simulink model "precisionLanding"  (R2021b)
settings: Solver=VariableStepAuto  StartTime=0.0  StopTime=10.0  RelTol=1e-3
values from neighbouring files (symbols this model uses):
  alpha0 = 0.01    [forces_moments.m]    (also in forces_moments_testing.m; omegaController.m; precisionLanding.m)
  D = diag([0 k1*k3 k4/d])    [airspeedController.m]    (also in forces_moments.m; forces_moments_testing.m; precisionLanding.m)
  G = [sin(alpha) 0 -cos(alpha);-cos(alpha)*tan(beta) 1 -sin(alpha)*tan(beta);         cos(alpha)/cos(beta) 0 sin(alpha)/cos(beta)]    [forces_moments.m]    (also in forces_moments_testing.m; precisionLanding.m = [sin(alpha) 0 -cos(alpha);-cos(alpha)*tan(beta) 1 -sin(alpha)
  gama = 1    [airspeedController.m]    (also in forces_moments.m; forces_moments_testing.m; precisionLanding.m)
  k_VI = 0.8    [airspeedController.m]    (also in forces_moments.m; forces_moments_testing.m; main_precision_landing.m; precisionLanding.m)
  k_VP = 0.5    [airspeedController.m]    (also in forces_moments.m; forces_moments_testing.m; main_precision_landing.m; precisionLanding.m)
  Maabb = [P.C_ell_beta 0; 0 P.C_m_alpha; P.C_n_beta 0]    [forces_moments.m]    (also in forces_moments_testing.m; omegaController.m; precisionLanding.m)
  mass = 25    [airspeedController.m]    (also in precisionLanding.m = P.mass)
  Mdd = [0,P.C_ell_delta_a,P.C_ell_delta_r ... (first row only)    [forces_moments.m]    (also in forces_moments_testing.m; omegaController.m; precisionLanding.m)
  Moo = Moo/(2*V)    [forces_moments.m]    (also in forces_moments_testing.m; omegaController.m; precisionLanding.m)
  w = x(6)    [forces_moments.m]    (also in forces_moments_testing.m)
undefined symbols (not defined in the file or in its folder): gravity
settings Model: Creator=pedro  LastModifiedBy=joaomoura
settings SolverCC: AlgebraicLoopSolver=TrustRegion
settings DebuggingCC: SFMachineParentedDataDiag=warning
settings SFSimCC: CustomCodeUndefinedFunction=UseInterfaceOnly

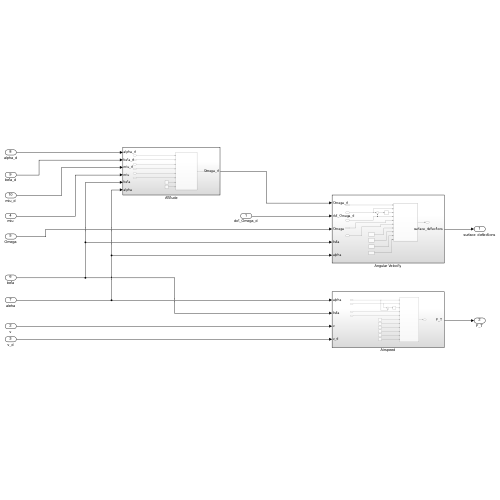
[thumbnail: Simulink's stored preview of the top-level diagram]
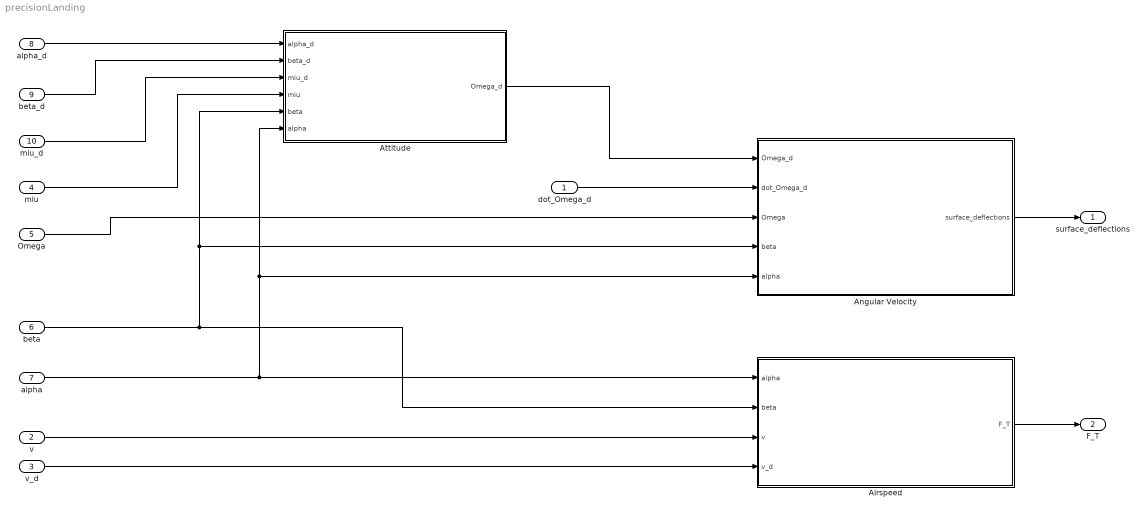
== system precisionLanding ==
  dot_Omega_d : Inport
  "v " : Inport  Port=2
  v_d : Inport  Port=3
  miu : Inport  Port=4
  "Omega " : Inport  Port=5
  beta : Inport  Port=6
  alpha : Inport  Port=7
  alpha_d : Inport  Port=8
  beta_d : Inport  Port=9
  miu_d : Inport  Port=10
  Airspeed : Subsystem
  Angular Velocity : Subsystem
  Attitude : Subsystem
  surface_deflections : Outport  VectorParamsAs1DForOutWhenUnconnected=off
  "F_T " : Outport  Port=2  VectorParamsAs1DForOutWhenUnconnected=off
  wires:
  Attitude/1(Omega_d) -> Angular Velocity/1(Omega_d)
  dot_Omega_d/1 -> Angular Velocity/2(dot_Omega_d)
  Angular Velocity/1(surface_deflections) -> surface_deflections/1
  "v "/1 -> Airspeed/3("v ")
  v_d/1 -> Airspeed/4(v_d)
  Airspeed/1("F_T ") -> "F_T "/1
  miu/1 -> Attitude/4(miu)
  alpha/1 -> Attitude/6(alpha), Angular Velocity/5(alpha), Airspeed/1(alpha)
  beta/1 -> Airspeed/2(beta), Attitude/5(beta), Angular Velocity/4(beta)
  "Omega "/1 -> Angular Velocity/3(Omega)
  alpha_d/1 -> Attitude/1(alpha_d)
  beta_d/1 -> Attitude/2(beta_d)
  miu_d/1 -> Attitude/3(miu_d)

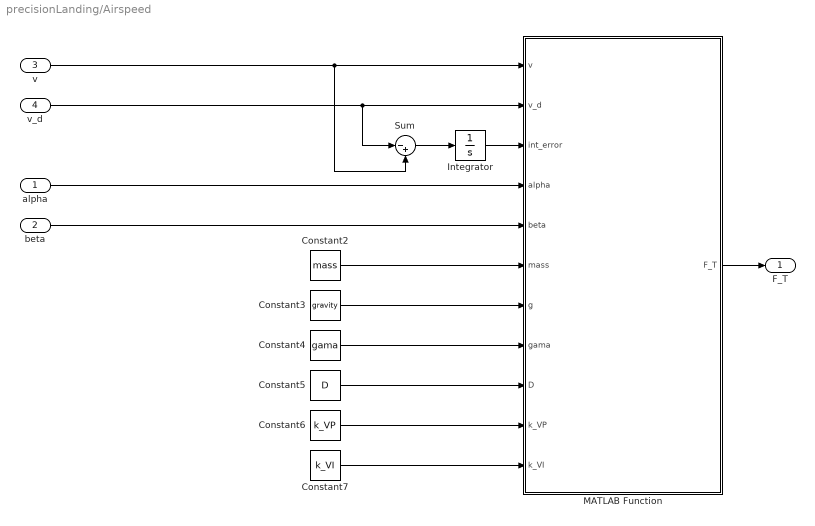
== system precisionLanding/Airspeed ==
  alpha : Inport
  beta : Inport  Port=2
  "v " : Inport  Port=3
  v_d : Inport  Port=4
  Constant2 : Constant  Value=mass
  Constant3 : Constant  Value=gravity
  Constant4 : Constant  Value=gama
  Constant5 : Constant  Value=D
  Constant6 : Constant  Value=k_VP
  Constant7 : Constant  Value=k_VI
  Integrator : Integrator
  MATLAB Function : MATLAB Function  TreatAsAtomicUnit=on
  Sum : Sum  Inputs=|-+
  "F_T " : Outport  VectorParamsAs1DForOutWhenUnconnected=off
  wires:
  Constant3/1 -> MATLAB Function/7(g)
  v_d/1 -> Sum/1, MATLAB Function/2(v_d)
  Constant4/1 -> MATLAB Function/8(gama)
  Constant7/1 -> MATLAB Function/11(k_VI)
  beta/1 -> MATLAB Function/5(beta)
  Constant5/1 -> MATLAB Function/9(D)
  Constant6/1 -> MATLAB Function/10(k_VP)
  MATLAB Function/1(F_T) -> "F_T "/1
  "v "/1 -> Sum/2, MATLAB Function/1(v)
  Integrator/1 -> MATLAB Function/3(int_error)
  alpha/1 -> MATLAB Function/4(alpha)
  Sum/1 -> Integrator/1
  Constant2/1 -> MATLAB Function/6(mass)

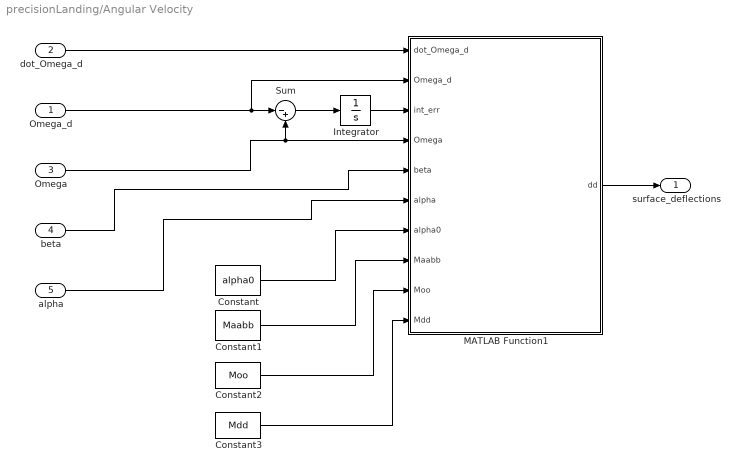
== system precisionLanding/Angular Velocity ==
  Omega_d : Inport
  dot_Omega_d : Inport  Port=2
  Omega : Inport  Port=3
  beta : Inport  Port=4
  alpha : Inport  Port=5
  Constant : Constant  Value=alpha0
  Constant1 : Constant  Value=Maabb
  Constant2 : Constant  Value=Moo
  Constant3 : Constant  Value=Mdd
  Integrator : Integrator
  MATLAB Function1 : MATLAB Function  TreatAsAtomicUnit=on
  Sum : Sum  Inputs=|-+
  surface_deflections : Outport  VectorParamsAs1DForOutWhenUnconnected=off
  wires:
  Constant1/1 -> MATLAB Function1/8(Maabb)
  Omega_d/1 -> MATLAB Function1/2(Omega_d), Sum/1
  Sum/1 -> Integrator/1
  Constant3/1 -> MATLAB Function1/10(Mdd)
  dot_Omega_d/1 -> MATLAB Function1/1(dot_Omega_d)
  beta/1 -> MATLAB Function1/5(beta)
  Omega/1 -> Sum/2, MATLAB Function1/4(Omega)
  Constant2/1 -> MATLAB Function1/9(Moo)
  Constant/1 -> MATLAB Function1/7(alpha0)
  Integrator/1 -> MATLAB Function1/3(int_err)
  MATLAB Function1/1(dd) -> surface_deflections/1
  alpha/1 -> MATLAB Function1/6(alpha)

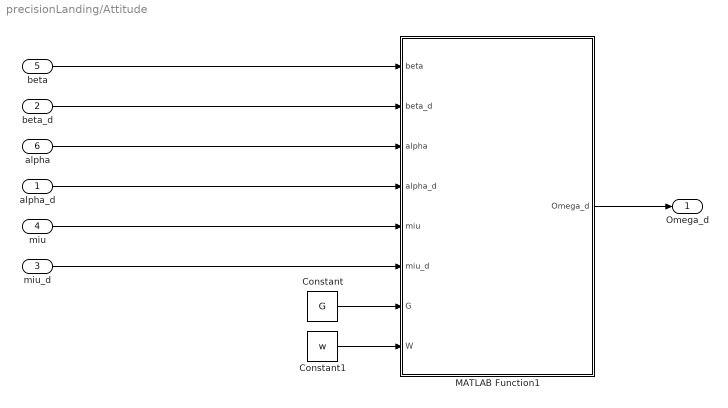
== system precisionLanding/Attitude ==
  alpha_d : Inport
  beta_d : Inport  Port=2
  miu_d : Inport  Port=3
  miu : Inport  Port=4
  beta : Inport  Port=5
  alpha : Inport  Port=6
  Constant : Constant  Value=G
  Constant1 : Constant  Value=w
  MATLAB Function1 : MATLAB Function  TreatAsAtomicUnit=on
  Omega_d : Outport  VectorParamsAs1DForOutWhenUnconnected=off
  wires:
  MATLAB Function1/1(Omega_d) -> Omega_d/1
  alpha_d/1 -> MATLAB Function1/4(alpha_d)
  beta_d/1 -> MATLAB Function1/2(beta_d)
  miu_d/1 -> MATLAB Function1/6(miu_d)
  miu/1 -> MATLAB Function1/5(miu)
  beta/1 -> MATLAB Function1/1(beta)
  alpha/1 -> MATLAB Function1/3(alpha)
  Constant/1 -> MATLAB Function1/7(G)
  Constant1/1 -> MATLAB Function1/8(W)

== matlab function precisionLanding/Angular Velocity/MATLAB Function1 ==
  data: dot_Omega_d input; Omega_d input; int_err input; Omega input; beta input; alpha input; alpha0 input; Maabb input; dd output; Moo input; Mdd input
function dd = controller(dot_Omega_d,Omega_d,int_err,Omega,beta,alpha,alpha0,Maabb,Moo,Mdd)
% Equation 48 [1]

    % gains
    kp = 1;
    ki = 1;
    
    % auxiliary calculations
    Soo = skew(Omega);
    
    % control law
    dd = Mdd\(Soo*Omega-...
        Maabb*[beta;alpha-alpha0]-...
        Moo*Omega-...
        kp*(Omega-Omega_d)-...
        ki*int_err+dot_Omega_d);
end

function S = skew(vector)
    S = [0,-vector(3),vector(2);
        vector(3),0,-vector(1);
        -vector(2),vector(1),0];
end

% [1] Serra, Pedro & Cunha, Rita & Hamel, T. & Silvestre, Carlos & Le Bras, Florent. (2015). Nonlinear Image-Based Visual Servo Controller for the Flare Maneuver of Fixed-Wing Aircraft Using Optical Flow. IEEE Transactions on Control Systems Technology. 23. 570–583. 10.1109/TCST.2014.2330996.

== matlab function precisionLanding/Airspeed/MATLAB Function ==
  data: v input; v_d input; F_T output; int_error input; alpha input; beta input; mass input; g input; gama input; D input; k_VP input; k_VI input
function F_T = airspeedController(v,v_d,int_error,alpha,beta,mass,g,gama,D,k_VP,k_VI)
% Equation 47 [1]

F_T = [(D + mass*g*sin(gama)/(cos(beta)*cos(alpha))] + ...
      [(k_VP*(v-v_d) + k_VI*int_error)/(cos(beta)*cos(alpha))];

end

% [1] Serra, Pedro & Cunha, Rita & Hamel, T. & Silvestre, Carlos & Le Bras, Florent. (2015). Nonlinear Image-Based Visual Servo Controller for the Flare Maneuver of Fixed-Wing Aircraft Using Optical Flow. IEEE Transactions on Control Systems Technology. 23. 570–583. 10.1109/TCST.2014.2330996.

== matlab function precisionLanding/Attitude/MATLAB Function1 ==
  data: beta input; beta_d input; alpha input; alpha_d input; miu input; miu_d input; G input; Omega_d output; W input
function Omega_d = controller(beta,beta_d,alpha,alpha_d,miu,miu_d, G, W)
    % gains
    Kp = 1;
    
    % control law
    Omega_d = inv(G)*(-W-Kp*[beta-beta_d;alpha-alpha_d;miu-miu_d];
end
